simulink model "STEVE_Simulation"  (R2025b)
settings: Solver=ode8  StartTime=0  StopTime=300  FixedStep=0.0001  MaxStep=0.0001  RelTol=1e-3
model workspace (MAT data in the model file):
  op_trim1 : opcond.OperatingReport (value not decoded)
undefined symbols (not defined in the file): a_gyro_fast, Actuators, AeroData, b_gyro_fast, C_inner_launch_d_Kd, C_inner_launch_d_Ki, C_inner_launch_d_Kp, C_inner_maxQ_d_Kd, C_inner_maxQ_d_Ki, C_inner_maxQ_d_Kp, C_inner_maxQ_d_Tf, C_outer_launch_d_Kd, C_outer_launch_d_Ki, C_outer_launch_d_Kp, C_outer_launch_d_N, C_outer_maxQ_d_Kd, C_outer_maxQ_d_Ki, C_outer_maxQ_d_Kp, dspblkCoreblockFVToolHelper, F, fractalcoef, fs_filter, fs_gyro, gcbh, Initial, K_gains, Light, max_q_margin, MIL, PrelookupData, Ref_Area, rocket_length, RocketAeroPhysical, time_vector, timeStep, Ts_inner, Ts_outer, wn_ramp
libraries: simulink x14, simulink_extras x11, slpidlib x10, aerolibwind2 x3, aerolibasang x3, aerolibtransform2 x2, aerolibatmos2 x1, sensorgpslib x1, mspsensorlib x1, aerolibconvert2 x1, aerolibactuator x1
(part 2 of 3)

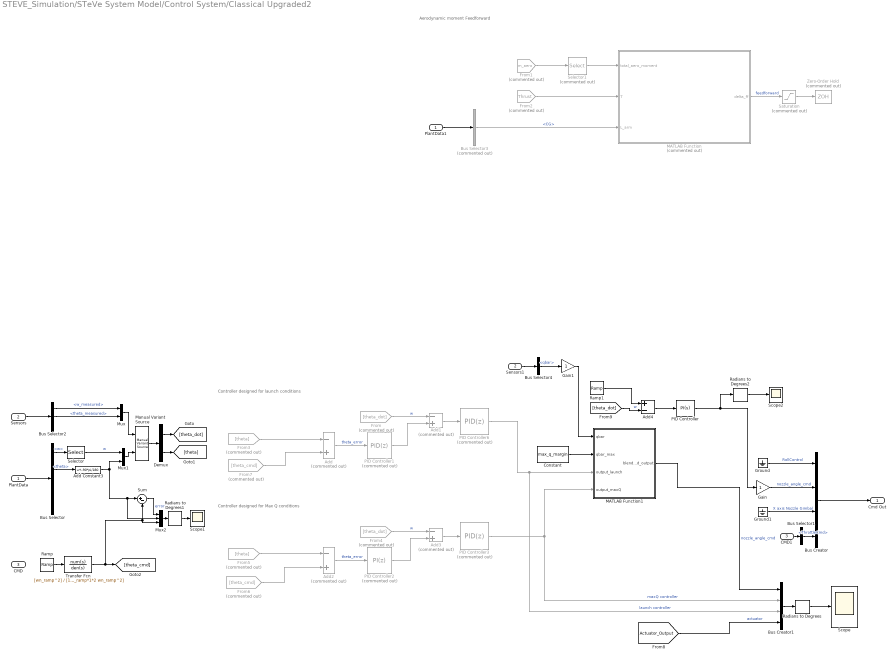
== system STEVE_Simulation/STeVe System Model/Control System/Classical Upgraded2 ==
  note: Controller designed for launch conditions
  note: Aerodynamic moment Feedforward
  note: Controller designed for Max Q conditions
  PlantData : Inport
  Sensors : Inport  Port=2
  CMD : Inport  Port=3
  Add{,1..3} (4 alike) : Sum  Commented=on  Inputs=-+
  Add Constant3 : Bias  Bias=-90*pi/180  SaturateOnIntegerOverflow=off
  Add4 : Sum  Inputs=+-
  Bus Creator : BusCreator  Inputs=4
  Bus Creator1 : BusCreator  Inputs=4
  Bus Selector : BusSelector  OutputSignals=w,body angles.theta,Ve,Xe
  Bus Selector1 : BusSelector  OutputSignals=ThrottleCmd
  Bus Selector2 : BusSelector  OutputSignals=w_measured,theta_measured,qbar
  Bus Selector3 : BusSelector  Commented=on  OutputSignals=CG
  Bus Selector4 : BusSelector  OutputSignals=qbar
  CMD1 : InportShadow  Port=3
  Constant : Constant  Value=max_q_margin
  Demux : Demux  Outputs=2
  From : From  Commented=on  GotoTag=theta_dot
  From1 : From  Commented=on  GotoTag=m_aero  TagVisibility=global
  From2 : From  Commented=on  GotoTag=Thrust  TagVisibility=global
  From3 : From  Commented=on  GotoTag=theta
  From4 : From  Commented=on  GotoTag=theta_dot
  From5 : From  Commented=on  GotoTag=theta
  From6 : From  Commented=on  GotoTag=theta_cmd
  From7 : From  Commented=on  GotoTag=theta_cmd
  Gain : Gain
  Gain1 : Gain
  Ground : Ground
  Ground1 : Ground
  MATLAB Function : MATLAB Function  Commented=on  TreatAsAtomicUnit=on
  MATLAB Function1 : MATLAB Function  TreatAsAtomicUnit=on
  Manual Variant Source : simulink/Signal Routing/Manual Variant Source  NumChoices=2  LabelModeActiveChoice=V_2
  Mux : Mux  Inputs=2
  Mux1 : Mux  Inputs=2
  Mux2 : Mux  Inputs=3
  PID Controller : slpidlib/PID Controller  Controller=PI  Form=Parallel  TimeDomain=Continuous-time  UseExternalTs=off  SampleTime=1/10  IntegratorMethod=Trapezoidal  FilterMethod=Forward Euler  ControllerParametersSource=internal  P=1.8265  I=14.0169  UseKiTs=off  D=0  UseExternalDerivativeSource=off  N=100  UseFilter=on  TunerSelectOption=Transfer Function Based (PID Tuner App)  InitialConditionSource=internal  InitialConditionForIntegrator=0  InitialConditionForFilter=0  DifferentiatorICPrevScaledInput=0  ExternalReset=none  TrackingMode=off  Kt=1  LimitOutput=off  SatLimitsSource=internal  UpperSaturationLimit=inf  LowerSaturationLimit=-inf  LinearizeAsGain=on  AntiWindupMode=none  Kb=1  LimitIntegrator=off  UpperIntegratorSaturationLimit=inf  LowerIntegratorSaturationLimit=-inf  POutMin=[]  POutMax=[]  IOutMin=[]  IOutMax=[]  DOutMin=[]  DOutMax=[]  NOutMin=[]  NOutMax=[]  SumOutMin=[]  SumOutMax=[]  SaturationOutMin=[]  SaturationOutMax=[]  PParamMin=[]  PParamMax=[]  IParamMin=[]  IParamMax=[]  DParamMin=[]  DParamMax=[]  NParamMin=[]  NParamMax=[]  KbParamMin=[]  KbParamMax=[]  KtParamMin=[]  KtParamMax=[]  KbOutMin=[]  KbOutMax=[]  KtOutMin=[]  KtOutMax=[]  IntegratorOutMin=[]  IntegratorOutMax=[]  FilterOutMin=[]  FilterOutMax=[]  SumI1OutMin=[]  SumI1OutMax=[]  SumI2OutMin=[]  SumI2OutMax=[]  SumI3OutMin=[]  SumI3OutMax=[]  SumI4OutMin=[]  SumI4OutMax=[]  SumDOutMin=[]  SumDOutMax=[]  DifferentiatorOutMin=[]  DifferentiatorOutMax=[]  FilterDiffOutCoefMin=[]  FilterDiffOutCoefMax=[]  ReciprocalOutMin=[]  ReciprocalOutMax=[]  SumDenOutMin=[]  SumDenOutMax=[]  SumNumOutMin=[]  SumNumOutMax=[]  DivideOutMin=[]  DivideOutMax=[]  UdiffTsProdOutMin=[]  UdiffTsProdOutMax=[]  NTsProdOutMin=[]  NTsProdOutMax=[]  UintegralTsProdOutMin=[]  UintegralTsProdOutMax=[]  UngainTsProdOutMin=[]  UngainTsProdOutMax=[]  ClampingZeroOutDataTypeStr=Inherit: Inherit via back propagation  ClampingZeroOutMin=[]  ClampingZeroOutMax=[]  FilterDenConstantOutDataTypeStr=Inherit: Inherit via back propagation  FilterDenConstantOutMin=[]  FilterDenConstantOutMax=[]  PCopyOutDataTypeStr=Inherit: Inherit via back propagation  PCopyOutMin=[]  PCopyOutMax=[]  NCopyOutDataTypeStr=Inherit: Inherit via back propagation  NCopyOutMin=[]  NCopyOutMax=[]  IntegratorContinuousStateAttributes=''  IntegratorStateMustResolveToSignalObject=off  IntegratorRTWStateStorageClass=Auto  FilterContinuousStateAttributes=''  FilterStateMustResolveToSignalObject=off  FilterRTWStateStorageClass=Auto  ParallelPVariant=InternalParameters  IdealPVariant=Disabled  IVariant=InternalParameters  DVariant=Disabled  IntegratorVariant=Continuous  SatVariant=Disabled  AWVariant=Passthrough  PCopyVariant=Disabled  TRVariant=Disabled  FdbkBlocksVariant=Forward  IdealPFdbkVariant=Disabled  SatFdbkVariant=Disabled  DerivativeFilterVariant=Disabled  NVariant=Disabled  NCopyVariant=Disabled_SignalSpec  FilterICVariant=Disabled  IntegratorICVariant=InternalICs  ExternalResetVariant=Disabled  TRSumVariant=Passthrough  SumFdbkVariant=Disabled  SumVariant=Sum_PI  TsampFilterVariant=InternalTs  TsampNgainVariant=Passthrough  TsampIntegralVariant=Disabled_SignalSpec  ExternalSaturationOutDataTypeStr=Inherit: Same as second input  DerivativeSourceVariant=Disabled  PreIntVariant=InternalPreInt
  PID Controller1 : slpidlib/PID Controller  Commented=on  Controller=PID  Form=Parallel  TimeDomain=Discrete-time  UseExternalTs=off  SampleTime=Ts_outer  IntegratorMethod=Forward Euler  FilterMethod=Forward Euler  ControllerParametersSource=internal  P=C_outer_launch_d_Kp  I=C_outer_launch_d_Ki  UseKiTs=off  D=C_outer_launch_d_Kd  UseExternalDerivativeSource=off  N=C_outer_launch_d_N  UseFilter=on  TunerSelectOption=Transfer Function Based (PID Tuner App)  InitialConditionSource=internal  InitialConditionForIntegrator=0  InitialConditionForFilter=0  DifferentiatorICPrevScaledInput=0  ExternalReset=none  TrackingMode=off  Kt=1  LimitOutput=off  SatLimitsSource=internal  UpperSaturationLimit=inf  LowerSaturationLimit=-inf  LinearizeAsGain=on  AntiWindupMode=none  Kb=1  LimitIntegrator=off  UpperIntegratorSaturationLimit=inf  LowerIntegratorSaturationLimit=-inf  POutMin=[]  POutMax=[]  IOutMin=[]  IOutMax=[]  DOutMin=[]  DOutMax=[]  NOutMin=[]  NOutMax=[]  SumOutMin=[]  SumOutMax=[]  SaturationOutMin=[]  SaturationOutMax=[]  PParamMin=[]  PParamMax=[]  IParamMin=[]  IParamMax=[]  DParamMin=[]  DParamMax=[]  NParamMin=[]  NParamMax=[]  KbParamMin=[]  KbParamMax=[]  KtParamMin=[]  KtParamMax=[]  KbOutMin=[]  KbOutMax=[]  KtOutMin=[]  KtOutMax=[]  IntegratorOutMin=[]  IntegratorOutMax=[]  FilterOutMin=[]  FilterOutMax=[]  SumI1OutMin=[]  SumI1OutMax=[]  SumI2OutMin=[]  SumI2OutMax=[]  SumI3OutMin=[]  SumI3OutMax=[]  SumI4OutMin=[]  SumI4OutMax=[]  SumDOutMin=[]  SumDOutMax=[]  DifferentiatorOutMin=[]  DifferentiatorOutMax=[]  FilterDiffOutCoefMin=[]  FilterDiffOutCoefMax=[]  ReciprocalOutMin=[]  ReciprocalOutMax=[]  SumDenOutMin=[]  SumDenOutMax=[]  SumNumOutMin=[]  SumNumOutMax=[]  DivideOutMin=[]  DivideOutMax=[]  UdiffTsProdOutMin=[]  UdiffTsProdOutMax=[]  NTsProdOutMin=[]  NTsProdOutMax=[]  UintegralTsProdOutMin=[]  UintegralTsProdOutMax=[]  UngainTsProdOutMin=[]  UngainTsProdOutMax=[]  ClampingZeroOutDataTypeStr=Inherit: Inherit via back propagation  ClampingZeroOutMin=[]  ClampingZeroOutMax=[]  FilterDenConstantOutDataTypeStr=Inherit: Inherit via back propagation  FilterDenConstantOutMin=[]  FilterDenConstantOutMax=[]  PCopyOutDataTypeStr=Inherit: Inherit via back propagation  PCopyOutMin=[]  PCopyOutMax=[]  NCopyOutDataTypeStr=Inherit: Inherit via back propagation  NCopyOutMin=[]  NCopyOutMax=[]  IntegratorContinuousStateAttributes=''  IntegratorStateMustResolveToSignalObject=off  IntegratorRTWStateStorageClass=Auto  FilterContinuousStateAttributes=''  FilterStateMustResolveToSignalObject=off  FilterRTWStateStorageClass=Auto  ParallelPVariant=InternalParameters  IdealPVariant=Disabled  IVariant=InternalParameters  DVariant=InternalParameters  IntegratorVariant=Discrete  SatVariant=Disabled  AWVariant=Passthrough  PCopyVariant=Disabled  TRVariant=Disabled  FdbkBlocksVariant=Forward  IdealPFdbkVariant=Disabled  SatFdbkVariant=Disabled  DerivativeFilterVariant=ForwardEulerFilter  NVariant=InternalParameters  NCopyVariant=Disabled  FilterICVariant=InternalICsFilter  IntegratorICVariant=InternalICs  ExternalResetVariant=Disabled  TRSumVariant=Passthrough  SumFdbkVariant=Disabled  SumVariant=Sum_PID  TsampFilterVariant=InternalTs  TsampNgainVariant=Passthrough  TsampIntegralVariant=Disabled_SignalSpec  ExternalSaturationOutDataTypeStr=Inherit: Same as second input  DerivativeSourceVariant=ErrorSignal  PreIntVariant=InternalPreInt
  PID Controller2 : slpidlib/PID Controller  Commented=on  Controller=PI  Form=Parallel  TimeDomain=Discrete-time  UseExternalTs=off  SampleTime=Ts_outer  IntegratorMethod=Forward Euler  FilterMethod=Forward Euler  ControllerParametersSource=internal  P=C_outer_maxQ_d_Kp  I=C_outer_maxQ_d_Ki  UseKiTs=off  D=C_outer_maxQ_d_Kd  UseExternalDerivativeSource=off  N=3.44088549948957  UseFilter=off  TunerSelectOption=Transfer Function Based (PID Tuner App)  InitialConditionSource=internal  InitialConditionForIntegrator=0  InitialConditionForFilter=0  DifferentiatorICPrevScaledInput=0  ExternalReset=none  TrackingMode=off  Kt=1  LimitOutput=off  SatLimitsSource=internal  UpperSaturationLimit=inf  LowerSaturationLimit=-inf  LinearizeAsGain=on  AntiWindupMode=none  Kb=1  LimitIntegrator=off  UpperIntegratorSaturationLimit=inf  LowerIntegratorSaturationLimit=-inf  POutMin=[]  POutMax=[]  IOutMin=[]  IOutMax=[]  DOutMin=[]  DOutMax=[]  NOutMin=[]  NOutMax=[]  SumOutMin=[]  SumOutMax=[]  SaturationOutMin=[]  SaturationOutMax=[]  PParamMin=[]  PParamMax=[]  IParamMin=[]  IParamMax=[]  DParamMin=[]  DParamMax=[]  NParamMin=[]  NParamMax=[]  KbParamMin=[]  KbParamMax=[]  KtParamMin=[]  KtParamMax=[]  KbOutMin=[]  KbOutMax=[]  KtOutMin=[]  KtOutMax=[]  IntegratorOutMin=[]  IntegratorOutMax=[]  FilterOutMin=[]  FilterOutMax=[]  SumI1OutMin=[]  SumI1OutMax=[]  SumI2OutMin=[]  SumI2OutMax=[]  SumI3OutMin=[]  SumI3OutMax=[]  SumI4OutMin=[]  SumI4OutMax=[]  SumDOutMin=[]  SumDOutMax=[]  DifferentiatorOutMin=[]  DifferentiatorOutMax=[]  FilterDiffOutCoefMin=[]  FilterDiffOutCoefMax=[]  ReciprocalOutMin=[]  ReciprocalOutMax=[]  SumDenOutMin=[]  SumDenOutMax=[]  SumNumOutMin=[]  SumNumOutMax=[]  DivideOutMin=[]  DivideOutMax=[]  UdiffTsProdOutMin=[]  UdiffTsProdOutMax=[]  NTsProdOutMin=[]  NTsProdOutMax=[]  UintegralTsProdOutMin=[]  UintegralTsProdOutMax=[]  UngainTsProdOutMin=[]  UngainTsProdOutMax=[]  ClampingZeroOutDataTypeStr=Inherit: Inherit via back propagation  ClampingZeroOutMin=[]  ClampingZeroOutMax=[]  FilterDenConstantOutDataTypeStr=Inherit: Inherit via back propagation  FilterDenConstantOutMin=[]  FilterDenConstantOutMax=[]  PCopyOutDataTypeStr=Inherit: Inherit via back propagation  PCopyOutMin=[]  PCopyOutMax=[]  NCopyOutDataTypeStr=Inherit: Inherit via back propagation  NCopyOutMin=[]  NCopyOutMax=[]  IntegratorContinuousStateAttributes=''  IntegratorStateMustResolveToSignalObject=off  IntegratorRTWStateStorageClass=Auto  FilterContinuousStateAttributes=''  FilterStateMustResolveToSignalObject=off  FilterRTWStateStorageClass=Auto  ParallelPVariant=InternalParameters  IdealPVariant=Disabled  IVariant=InternalParameters  DVariant=Disabled  IntegratorVariant=Discrete  SatVariant=Disabled  AWVariant=Passthrough  PCopyVariant=Disabled  TRVariant=Disabled  FdbkBlocksVariant=Forward  IdealPFdbkVariant=Disabled  SatFdbkVariant=Disabled  DerivativeFilterVariant=Disabled  NVariant=Disabled  NCopyVariant=Disabled_SignalSpec  FilterICVariant=Disabled  IntegratorICVariant=InternalICs  ExternalResetVariant=Disabled  TRSumVariant=Passthrough  SumFdbkVariant=Disabled  SumVariant=Sum_PI  TsampFilterVariant=InternalTs  TsampNgainVariant=Passthrough  TsampIntegralVariant=Disabled_SignalSpec  ExternalSaturationOutDataTypeStr=Inherit: Same as second input  DerivativeSourceVariant=Disabled  PreIntVariant=InternalPreInt
  PID Controller3 : slpidlib/PID Controller  Commented=on  Controller=PID  Form=Parallel  TimeDomain=Discrete-time  UseExternalTs=off  SampleTime=Ts_inner  IntegratorMethod=Forward Euler  FilterMethod=Forward Euler  ControllerParametersSource=internal  P=C_inner_maxQ_d_Kp  I=C_inner_maxQ_d_Ki  UseKiTs=off  D=C_inner_maxQ_d_Kd  UseExternalDerivativeSource=off  N=C_inner_maxQ_d_Tf  UseFilter=on  TunerSelectOption=Transfer Function Based (PID Tuner App)  InitialConditionSource=internal  InitialConditionForIntegrator=0  InitialConditionForFilter=0  DifferentiatorICPrevScaledInput=0  ExternalReset=none  TrackingMode=off  Kt=1  LimitOutput=on  SatLimitsSource=internal  UpperSaturationLimit=10*pi/180  LowerSaturationLimit=-10*pi/180  LinearizeAsGain=on  AntiWindupMode=clamping  Kb=1  LimitIntegrator=on  UpperIntegratorSaturationLimit=10*pi/180  LowerIntegratorSaturationLimit=-10*pi/180  POutMin=[]  POutMax=[]  IOutMin=[]  IOutMax=[]  DOutMin=[]  DOutMax=[]  NOutMin=[]  NOutMax=[]  SumOutMin=[]  SumOutMax=[]  SaturationOutMin=[]  SaturationOutMax=[]  PParamMin=[]  PParamMax=[]  IParamMin=[]  IParamMax=[]  DParamMin=[]  DParamMax=[]  NParamMin=[]  NParamMax=[]  KbParamMin=[]  KbParamMax=[]  KtParamMin=[]  KtParamMax=[]  KbOutMin=[]  KbOutMax=[]  KtOutMin=[]  KtOutMax=[]  IntegratorOutMin=[]  IntegratorOutMax=[]  FilterOutMin=[]  FilterOutMax=[]  SumI1OutMin=[]  SumI1OutMax=[]  SumI2OutMin=[]  SumI2OutMax=[]  SumI3OutMin=[]  SumI3OutMax=[]  SumI4OutMin=[]  SumI4OutMax=[]  SumDOutMin=[]  SumDOutMax=[]  DifferentiatorOutMin=[]  DifferentiatorOutMax=[]  FilterDiffOutCoefMin=[]  FilterDiffOutCoefMax=[]  ReciprocalOutMin=[]  ReciprocalOutMax=[]  SumDenOutMin=[]  SumDenOutMax=[]  SumNumOutMin=[]  SumNumOutMax=[]  DivideOutMin=[]  DivideOutMax=[]  UdiffTsProdOutMin=[]  UdiffTsProdOutMax=[]  NTsProdOutMin=[]  NTsProdOutMax=[]  UintegralTsProdOutMin=[]  UintegralTsProdOutMax=[]  UngainTsProdOutMin=[]  UngainTsProdOutMax=[]  ClampingZeroOutDataTypeStr=Inherit: Inherit via back propagation  ClampingZeroOutMin=[]  ClampingZeroOutMax=[]  FilterDenConstantOutDataTypeStr=Inherit: Inherit via back propagation  FilterDenConstantOutMin=[]  FilterDenConstantOutMax=[]  PCopyOutDataTypeStr=Inherit: Inherit via back propagation  PCopyOutMin=[]  PCopyOutMax=[]  NCopyOutDataTypeStr=Inherit: Inherit via back propagation  NCopyOutMin=[]  NCopyOutMax=[]  IntegratorContinuousStateAttributes=''  IntegratorStateMustResolveToSignalObject=off  IntegratorRTWStateStorageClass=Auto  FilterContinuousStateAttributes=''  FilterStateMustResolveToSignalObject=off  FilterRTWStateStorageClass=Auto  ParallelPVariant=InternalParameters  IdealPVariant=Disabled  IVariant=InternalParameters  DVariant=InternalParameters  IntegratorVariant=Discrete  SatVariant=Enabled  AWVariant=DiscClampingParallel  PCopyVariant=Disabled  TRVariant=Disabled  FdbkBlocksVariant=Forward  IdealPFdbkVariant=Disabled  SatFdbkVariant=Disabled  DerivativeFilterVariant=ForwardEulerFilter  NVariant=InternalParameters  NCopyVariant=Disabled  FilterICVariant=InternalICsFilter  IntegratorICVariant=InternalICs  ExternalResetVariant=Disabled  TRSumVariant=Passthrough  SumFdbkVariant=Disabled  SumVariant=Sum_PID  TsampFilterVariant=InternalTs  TsampNgainVariant=Passthrough  TsampIntegralVariant=Disabled_SignalSpec  ExternalSaturationOutDataTypeStr=Inherit: Same as second input  DerivativeSourceVariant=ErrorSignal  PreIntVariant=InternalPreInt
  PID Controller6 : slpidlib/PID Controller  Commented=on  Controller=PID  Form=Parallel  TimeDomain=Discrete-time  UseExternalTs=off  SampleTime=Ts_inner  IntegratorMethod=Forward Euler  FilterMethod=Forward Euler  ControllerParametersSource=internal  P=C_inner_launch_d_Kp  I=C_inner_launch_d_Ki  UseKiTs=off  D=C_inner_launch_d_Kd  UseExternalDerivativeSource=off  N=100  UseFilter=off  TunerSelectOption=Transfer Function Based (PID Tuner App)  InitialConditionSource=internal  InitialConditionForIntegrator=0  InitialConditionForFilter=0  DifferentiatorICPrevScaledInput=0  ExternalReset=none  TrackingMode=off  Kt=1  LimitOutput=on  SatLimitsSource=internal  UpperSaturationLimit=10*pi/180  LowerSaturationLimit=-10*pi/180  LinearizeAsGain=on  AntiWindupMode=clamping  Kb=1  LimitIntegrator=on  UpperIntegratorSaturationLimit=10*pi/180  LowerIntegratorSaturationLimit=-10*pi/180  POutMin=[]  POutMax=[]  IOutMin=[]  IOutMax=[]  DOutMin=[]  DOutMax=[]  NOutMin=[]  NOutMax=[]  SumOutMin=[]  SumOutMax=[]  SaturationOutMin=[]  SaturationOutMax=[]  PParamMin=[]  PParamMax=[]  IParamMin=[]  IParamMax=[]  DParamMin=[]  DParamMax=[]  NParamMin=[]  NParamMax=[]  KbParamMin=[]  KbParamMax=[]  KtParamMin=[]  KtParamMax=[]  KbOutMin=[]  KbOutMax=[]  KtOutMin=[]  KtOutMax=[]  IntegratorOutMin=[]  IntegratorOutMax=[]  FilterOutMin=[]  FilterOutMax=[]  SumI1OutMin=[]  SumI1OutMax=[]  SumI2OutMin=[]  SumI2OutMax=[]  SumI3OutMin=[]  SumI3OutMax=[]  SumI4OutMin=[]  SumI4OutMax=[]  SumDOutMin=[]  SumDOutMax=[]  DifferentiatorOutMin=[]  DifferentiatorOutMax=[]  FilterDiffOutCoefMin=[]  FilterDiffOutCoefMax=[]  ReciprocalOutMin=[]  ReciprocalOutMax=[]  SumDenOutMin=[]  SumDenOutMax=[]  SumNumOutMin=[]  SumNumOutMax=[]  DivideOutMin=[]  DivideOutMax=[]  UdiffTsProdOutMin=[]  UdiffTsProdOutMax=[]  NTsProdOutMin=[]  NTsProdOutMax=[]  UintegralTsProdOutMin=[]  UintegralTsProdOutMax=[]  UngainTsProdOutMin=[]  UngainTsProdOutMax=[]  ClampingZeroOutDataTypeStr=Inherit: Inherit via back propagation  ClampingZeroOutMin=[]  ClampingZeroOutMax=[]  FilterDenConstantOutDataTypeStr=Inherit: Inherit via back propagation  FilterDenConstantOutMin=[]  FilterDenConstantOutMax=[]  PCopyOutDataTypeStr=Inherit: Inherit via back propagation  PCopyOutMin=[]  PCopyOutMax=[]  NCopyOutDataTypeStr=Inherit: Inherit via back propagation  NCopyOutMin=[]  NCopyOutMax=[]  IntegratorContinuousStateAttributes=''  IntegratorStateMustResolveToSignalObject=off  IntegratorRTWStateStorageClass=Auto  FilterContinuousStateAttributes=''  FilterStateMustResolveToSignalObject=off  FilterRTWStateStorageClass=Auto  ParallelPVariant=InternalParameters  IdealPVariant=Disabled  IVariant=InternalParameters  DVariant=InternalParameters  IntegratorVariant=Discrete  SatVariant=Enabled  AWVariant=DiscClampingParallel  PCopyVariant=Disabled  TRVariant=Disabled  FdbkBlocksVariant=Forward  IdealPFdbkVariant=Disabled  SatFdbkVariant=Disabled  DerivativeFilterVariant=Differentiator  NVariant=Passthrough  NCopyVariant=Disabled_SignalSpec  FilterICVariant=InternalICsDifferentiator  IntegratorICVariant=InternalICs  ExternalResetVariant=Disabled  TRSumVariant=Passthrough  SumFdbkVariant=Disabled  SumVariant=Sum_PID  TsampFilterVariant=InternalTs  TsampNgainVariant=Passthrough  TsampIntegralVariant=Disabled_SignalSpec  ExternalSaturationOutDataTypeStr=Inherit: Same as second input  DerivativeSourceVariant=ErrorSignal  PreIntVariant=InternalPreInt
  PlantData1 : InportShadow
  Radians to Degrees : simulink_extras/Transformations/Radians to Degrees
  Radians to Degrees1 : simulink_extras/Transformations/Radians to Degrees
  Radians to Degrees2 : simulink_extras/Transformations/Radians to Degrees
  Ramp : simulink/Sources/Ramp  slope=-(50/60)*pi/180  start=0  InitialOutput=0
  Ramp1 : simulink/Sources/Ramp  slope=0  start=0  InitialOutput=0
  Saturation : Saturate  Commented=on  UpperLimit=10*pi/180  LowerLimit=-10*pi/180
  Scope : Scope
      settings: ActiveDisplayYMinimum=-0.083485750616447252  ActiveDisplayYMaximum=2.7048040540539371  DataLoggingVariableName=ScopeData3
  Scope1 : Scope
      settings: ActiveDisplayYMinimum=-44.397461498284216  ActiveDisplayYMaximum=2.337544107445984  DataLoggingVariableName=ScopeData4
  Scope2 : Scope
      settings: ActiveDisplayYMinimum=-0.57661888935781047  ActiveDisplayYMaximum=0.0662657690157187  DataLoggingVariableName=ScopeData9
  Selector : Selector  InputPortWidth=3  IndexOptions=Index vector (dialog)  Indices=[2]  OutputSizes=1
  Selector1 : Selector  Commented=on  InputPortWidth=3  IndexOptions=Index vector (dialog)  Indices=[2]  OutputSizes=1
  Sensors1 : InportShadow  Port=2
  Sum : Sum  Inputs=|+-
  Transfer Fcn : TransferFcn  Numerator=[wn_ramp^2]  Denominator=[1 wn_ramp*1*2 wn_ramp^2]
  Zero-Order Hold : ZeroOrderHold  Commented=on  SampleTime=0.005
  Cmd Out : Outport
  wires:
  Selector1/1 -> MATLAB Function/1(total_aero_moment)
  PlantData/1 -> Bus Selector/1
  From1/1 -> Selector1/1
  Bus Selector/1 -> Selector/1  "<w>"
  Ground1/1 -> Bus Creator/3  "X axis Nozzle Gimbal"
  Bus Selector3/1 -> MATLAB Function/3(L_arm)  "<CG>"
  Gain/1 -> Bus Creator/2  "nozzle_angle_cmd"
  MATLAB Function/1(delta_ff) -> Saturation/1  "feedforward"
  From/1 -> Add1/1  "w"
  PlantData1/1 -> Bus Selector3/1
  From7/1 -> Add/2
  Ground/1 -> Bus Creator/1  "RollControl"
  From2/1 -> MATLAB Function/2(T)
  Bus Creator/1 -> Cmd Out/1
  Add/1 -> PID Controller1/1  "theta_error"
  PID Controller6/1 -> Bus Creator1/3, MATLAB Function1/3(output_launch)  "launch controller"
  Add1/1 -> PID Controller6/1
  Sensors/1 -> Bus Selector2/1
  Saturation/1 -> Zero-Order Hold/1
  From3/1 -> Add/1
  CMD1/1 -> Bus Selector1/1
  Bus Selector1/1 -> Bus Creator/4  "<ThrottleCmd>"
  PID Controller1/1 -> Add1/2
  Bus Selector/2 -> Add Constant3/1  "<theta>"
  Add2/1 -> PID Controller2/1  "theta_error"
  From5/1 -> Add2/1
  Add3/1 -> PID Controller3/1
  PID Controller3/1 -> Bus Creator1/2, MATLAB Function1/4(output_maxQ)  "maxQ controller"
  PID Controller2/1 -> Add3/2
  From6/1 -> Add2/2
  From4/1 -> Add3/1  "w"
  Ramp/1 -> Transfer Fcn/1
  Sensors1/1 -> Bus Selector4/1
  MATLAB Function1/1(blended_output) -> Bus Creator1/1  "nozzle_angle_cmd"
  Constant/1 -> MATLAB Function1/2(qbar_max)
  Bus Selector4/1 -> Gain1/1  "<qbar>"
  [Actuator_Output] -> Bus Creator1/4  "actuator"
  Transfer Fcn/1 -> Mux2/3, Sum/2, [theta_cmd]
  Bus Selector2/1 -> Mux/1  "<w_measured>"
  Bus Selector2/2 -> Mux/2  "<theta_measured>"
  Mux/1 -> Manual Variant Source/1
  Manual Variant Source/1 -> Demux/1
  Demux/1 -> [theta_dot]
  Demux/2 -> [theta]
  Selector/1 -> Mux1/1  "w"
  Mux1/1 -> Manual Variant Source/2
  Add Constant3/1 -> Mux2/2, Sum/1, Mux1/2
  Sum/1 -> Mux2/1  "error"
  Gain1/1 -> MATLAB Function1/1(qbar)
  Bus Creator1/1 -> Radians to Degrees/1
  Radians to Degrees/1 -> Scope/1
  Mux2/1 -> Radians to Degrees1/1
  Radians to Degrees1/1 -> Scope1/1
  [theta_dot] -> Add4/2  "w"
  Add4/1 -> PID Controller/1
  Ramp1/1 -> Add4/1
  PID Controller/1 -> Radians to Degrees2/1, Gain/1
  Radians to Degrees2/1 -> Scope2/1

== system STEVE_Simulation/STeVe System Model/Control System/ControlSystem Classical ==
  note: FeedForward Controller
  AvionicsBus : Inport
  Guidance : Inport  Port=2
  Add : Sum
  Bus Creator : BusCreator  Inputs=4
  Bus Selector : BusSelector  OutputSignals=ThetaCmd,ThrottleCmd
  Bus Selector1 : BusSelector  OutputSignals=w,body angles.theta
  Constant : Constant  Value=Actuators.Engine.MaxThrust
  Constant1 : Constant  Value=4
  Ground : Ground
  Ground1 : Ground
  Integrator : Integrator
  Multiply : Gain
  Multiply1 : Gain  Gain=0.1
  Multiply2 : Gain  Gain=-1
  Multiply3 : Gain
  Multiply4 : Gain  Gain=0.05
  Product : Product
  Product1 : Product  Inputs=*/
  Selector : Selector  InputPortWidth=3  IndexOptions=Index vector (dialog)  Indices=2  OutputSizes=1
  Selector1 : Selector  InputPortWidth=3  IndexOptions=Index vector (dialog)  Indices=[2]  OutputSizes=1
  Sum : Sum  Inputs=-+|
  Sum1 : Sum  Inputs=-|+|+
  Sum2 : Sum  Inputs=|++
  cmd : Outport
  wires:
  Bus Creator/1 -> cmd/1
  Ground/1 -> Bus Creator/1  "RollControl"
  Ground1/1 -> Bus Creator/3  "X axis Nozzle Gimbal"
  Guidance/1 -> Bus Selector/1
  Bus Selector/2 -> Bus Creator/4  "<ThrottleCmd>"
  Bus Selector/1 -> Sum/2  "<ThetaCmd>"
  AvionicsBus/1 -> Bus Selector1/1
  Bus Selector1/1 -> Selector/1  "<w>"
  Multiply/1 -> Bus Creator/2  "nozzle_angle_cmd"
  Sum1/1 -> Integrator/1, Multiply1/1  "thetadot_error"
  Selector/1 -> Sum1/1  "thetadot"
  Bus Selector1/2 -> Sum/1  "<theta>"
  Sum/1 -> Multiply3/1  "theta_error"
  Constant1/1 -> Product/2
  Constant/1 -> Product/1
  Product/1 -> Product1/2
  [m_aero] -> Selector1/1
  Selector1/1 -> Product1/1
  Add/1 -> Multiply/1  "total_nozzle_angle_rad"
  Product1/1 -> Multiply2/1
  Multiply3/1 -> Sum1/2  "pitch_controller_cmd"
  Sum2/1 -> Add/2  "pitchrate_controller_cmd"
  Multiply2/1 -> Add/1  "feedforward_cmd"
  Multiply1/1 -> Sum2/1
  Integrator/1 -> Multiply4/1
  Multiply4/1 -> Sum2/2

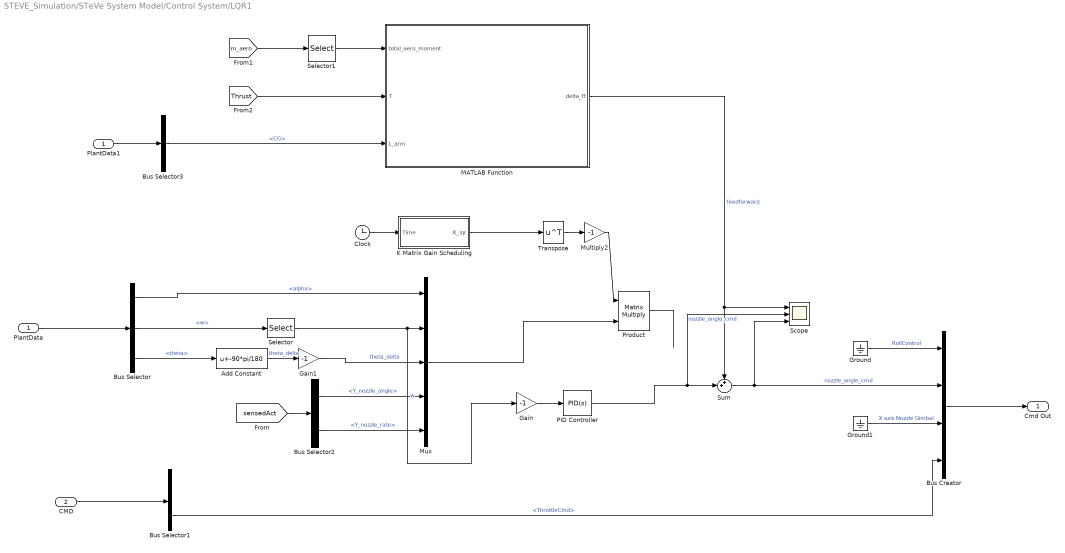
== system STEVE_Simulation/STeVe System Model/Control System/LQR1 ==
  PlantData : Inport
  CMD : Inport  Port=2
  Add Constant : Bias  Bias=-90*pi/180  SaturateOnIntegerOverflow=off
  Bus Creator : BusCreator  Inputs=4
  Bus Selector : BusSelector  OutputSignals=alpha,w,body angles.theta
  Bus Selector1 : BusSelector  OutputSignals=ThetaCmd,ThrottleCmd
  Bus Selector2 : BusSelector  OutputSignals=Y_nozzle_angle,Y_nozzle_rate
  Bus Selector3 : BusSelector  OutputSignals=CG
  Clock : Clock
  Gain : Gain  Gain=-1
  Gain1 : Gain  Gain=-1
  Ground : Ground
  Ground1 : Ground
  K Matrix Gain Scheduling : Subsystem
  MATLAB Function : MATLAB Function  TreatAsAtomicUnit=on
  Multiply2 : Gain  Gain=-1
  Mux : Mux  Inputs=5
  PID Controller : slpidlib/PID Controller  Controller=PID  Form=Parallel  TimeDomain=Continuous-time  UseExternalTs=off  SampleTime=-1  IntegratorMethod=Forward Euler  FilterMethod=Forward Euler  ControllerParametersSource=internal  P=0.00297430815475411  I=0.00270872553316802  UseKiTs=off  D=0.00015125727616714  UseExternalDerivativeSource=off  N=19.0953356399636  UseFilter=on  TunerSelectOption=Transfer Function Based (PID Tuner App)  InitialConditionSource=internal  InitialConditionForIntegrator=0  InitialConditionForFilter=0  DifferentiatorICPrevScaledInput=0  ExternalReset=none  TrackingMode=off  Kt=1  LimitOutput=off  SatLimitsSource=internal  UpperSaturationLimit=inf  LowerSaturationLimit=-inf  LinearizeAsGain=on  AntiWindupMode=none  Kb=1  LimitIntegrator=off  UpperIntegratorSaturationLimit=inf  LowerIntegratorSaturationLimit=-inf  POutMin=[]  POutMax=[]  IOutMin=[]  IOutMax=[]  DOutMin=[]  DOutMax=[]  NOutMin=[]  NOutMax=[]  SumOutMin=[]  SumOutMax=[]  SaturationOutMin=[]  SaturationOutMax=[]  PParamMin=[]  PParamMax=[]  IParamMin=[]  IParamMax=[]  DParamMin=[]  DParamMax=[]  NParamMin=[]  NParamMax=[]  KbParamMin=[]  KbParamMax=[]  KtParamMin=[]  KtParamMax=[]  KbOutMin=[]  KbOutMax=[]  KtOutMin=[]  KtOutMax=[]  IntegratorOutMin=[]  IntegratorOutMax=[]  FilterOutMin=[]  FilterOutMax=[]  SumI1OutMin=[]  SumI1OutMax=[]  SumI2OutMin=[]  SumI2OutMax=[]  SumI3OutMin=[]  SumI3OutMax=[]  SumI4OutMin=[]  SumI4OutMax=[]  SumDOutMin=[]  SumDOutMax=[]  DifferentiatorOutMin=[]  DifferentiatorOutMax=[]  FilterDiffOutCoefMin=[]  FilterDiffOutCoefMax=[]  ReciprocalOutMin=[]  ReciprocalOutMax=[]  SumDenOutMin=[]  SumDenOutMax=[]  SumNumOutMin=[]  SumNumOutMax=[]  DivideOutMin=[]  DivideOutMax=[]  UdiffTsProdOutMin=[]  UdiffTsProdOutMax=[]  NTsProdOutMin=[]  NTsProdOutMax=[]  UintegralTsProdOutMin=[]  UintegralTsProdOutMax=[]  UngainTsProdOutMin=[]  UngainTsProdOutMax=[]  ClampingZeroOutDataTypeStr=Inherit: Inherit via back propagation  ClampingZeroOutMin=[]  ClampingZeroOutMax=[]  FilterDenConstantOutDataTypeStr=Inherit: Inherit via back propagation  FilterDenConstantOutMin=[]  FilterDenConstantOutMax=[]  PCopyOutDataTypeStr=Inherit: Inherit via back propagation  PCopyOutMin=[]  PCopyOutMax=[]  NCopyOutDataTypeStr=Inherit: Inherit via back propagation  NCopyOutMin=[]  NCopyOutMax=[]  IntegratorContinuousStateAttributes=''  IntegratorStateMustResolveToSignalObject=off  IntegratorRTWStateStorageClass=Auto  FilterContinuousStateAttributes=''  FilterStateMustResolveToSignalObject=off  FilterRTWStateStorageClass=Auto  ParallelPVariant=InternalParameters  IdealPVariant=Disabled  IVariant=InternalParameters  DVariant=InternalParameters  IntegratorVariant=Continuous  SatVariant=Disabled  AWVariant=Passthrough  PCopyVariant=Disabled  TRVariant=Disabled  FdbkBlocksVariant=Forward  IdealPFdbkVariant=Disabled  SatFdbkVariant=Disabled  DerivativeFilterVariant=ContFilter  NVariant=InternalParameters  NCopyVariant=Disabled  FilterICVariant=InternalICsFilter  IntegratorICVariant=InternalICs  ExternalResetVariant=Disabled  TRSumVariant=Passthrough  SumFdbkVariant=Disabled  SumVariant=Sum_PID  TsampFilterVariant=InternalTs  TsampNgainVariant=Passthrough  TsampIntegralVariant=Disabled_SignalSpec  ExternalSaturationOutDataTypeStr=Inherit: Same as second input  DerivativeSourceVariant=ErrorSignal  PreIntVariant=InternalPreInt
  PlantData1 : InportShadow
  Product : Product  Multiplication=Matrix(*)
  Scope : Scope  NumInputPorts=3
      settings: ActiveDisplayYMinimum=-10.665603461907551  ActiveDisplayYMaximum=5.7104419346533186
  Selector : Selector  InputPortWidth=3  IndexOptions=Index vector (dialog)  Indices=[2]  OutputSizes=1
  Selector1 : Selector  InputPortWidth=3  IndexOptions=Index vector (dialog)  Indices=[2]  OutputSizes=1
  Sum : Sum  Inputs=++|
  Transpose : Math  Operator=transpose
  Cmd Out : Outport
  wires:
  PlantData/1 -> Bus Selector/1
  Bus Selector2/2 -> Mux/5  "<Y_nozzle_rate>"
  Ground/1 -> Bus Creator/1  "RollControl"
  Bus Selector/2 -> Selector/1  "<w>"
  Bus Selector2/1 -> Mux/4  "<Y_nozzle_angle>"
  [sensedAct] -> Bus Selector2/1
  Bus Selector1/2 -> Bus Creator/4  "<ThrottleCmd>"
  Bus Selector/1 -> Mux/1  "<alpha>"
  Mux/1 -> Product/2
  Ground1/1 -> Bus Creator/3  "X axis Nozzle Gimbal"
  Add Constant/1 -> Gain1/1  "theta_delta"
  Bus Creator/1 -> Cmd Out/1
  Selector/1 -> Gain/1, Mux/2  "w"
  CMD/1 -> Bus Selector1/1
  Bus Selector/3 -> Add Constant/1  "<theta>"
  K Matrix Gain Scheduling/1(K_lqr) -> Transpose/1
  Clock/1 -> K Matrix Gain Scheduling/1(Time)
  Transpose/1 -> Multiply2/1
  Multiply2/1 -> Product/1
  Sum/1 -> Scope/3, Bus Creator/2  "nozzle_angle_cmd"
  Gain1/1 -> Mux/3  "theta_delta"
  PlantData1/1 -> Bus Selector3/1
  Bus Selector3/1 -> MATLAB Function/3(L_arm)  "<CG>"
  [m_aero] -> Selector1/1
  [Thrust] -> MATLAB Function/2(T)
  Selector1/1 -> MATLAB Function/1(total_aero_moment)
  Product/1 -> ?
  MATLAB Function/1(delta_ff) -> Sum/1, Scope/1  "feedforward"
  PID Controller/1 -> Scope/2, Sum/2  "nozzle_angle_cmd"
  Gain/1 -> PID Controller/1

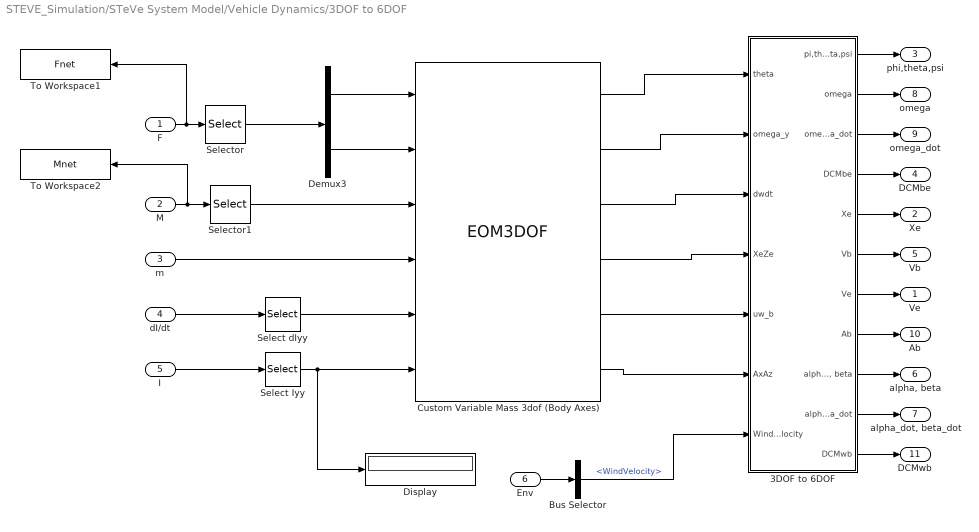
== system STEVE_Simulation/STeVe System Model/Vehicle Dynamics/3DOF to 6DOF ==
  F : Inport
  M : Inport  Port=2
  m : Inport  Port=3
  dI/dt : Inport  Port=4
  I : Inport  Port=5
  Env : Inport  Port=6
  3DOF to 6DOF : Subsystem
  Bus Selector : BusSelector  OutputSignals=WindVelocity
  Custom Variable Mass 3dof (Body Axes) : EOM3DOF  mtype=Custom Variable  v_ini=Initial.Conditions.V0  theta_ini=Initial.Conditions.theta0  pos_ini=[0 Initial.Conditions.h0]  g=0  vel_statename={'u','w'}  pos_statename={'Xe','Ze'}  q_statename='q'  theta_statename='theta'
  Demux3 : Demux  Outputs=2
  Display : Display
  Select Iyy : Selector  NumberOfDimensions=2  InputPortWidth=3  IndexOptions=Index vector (dialog),Index vector (dialog)  Indices=[2],[2]  OutputSizes=1,1
  Select dIyy : Selector  NumberOfDimensions=2  InputPortWidth=3  IndexOptions=Index vector (dialog),Index vector (dialog)  Indices=[2],[2]  OutputSizes=1,1
  Selector : Selector  InputPortWidth=3  IndexOptions=Index vector (dialog)  Indices=[1 3]  OutputSizes=1
  Selector1 : Selector  InputPortWidth=3  IndexOptions=Index vector (dialog)  Indices=[2]  OutputSizes=1
  To Workspace1 : ToWorkspace  VariableName=Fnet  SaveFormat=Timeseries  SampleTime=-1
  To Workspace2 : ToWorkspace  VariableName=Mnet  SaveFormat=Timeseries  SampleTime=-1
  Ve : Outport
  Xe : Outport  Port=2
  phi,theta,psi : Outport  Port=3
  DCMbe : Outport  Port=4
  Vb : Outport  Port=5
  "alpha, beta" : Outport  Port=6
  "alpha_dot, beta_dot" : Outport  Port=7
  omega : Outport  Port=8
  omega_dot : Outport  Port=9
  Ab : Outport  Port=10
  DCMwb : Outport  Port=11
  wires:
  F/1 -> To Workspace1/1, Selector/1
  Demux3/2 -> Custom Variable Mass 3dof (Body Axes)/2
  Demux3/1 -> Custom Variable Mass 3dof (Body Axes)/1
  Selector/1 -> Demux3/1
  M/1 -> To Workspace2/1, Selector1/1
  Selector1/1 -> Custom Variable Mass 3dof (Body Axes)/3
  Custom Variable Mass 3dof (Body Axes)/1 -> 3DOF to 6DOF/1(theta)
  Custom Variable Mass 3dof (Body Axes)/4 -> 3DOF to 6DOF/4(XeZe)
  Custom Variable Mass 3dof (Body Axes)/6 -> 3DOF to 6DOF/6(AxAz)
  3DOF to 6DOF/1(pi,theta,psi) -> phi,theta,psi/1
  3DOF to 6DOF/2(omega) -> omega/1
  3DOF to 6DOF/3(omega_dot) -> omega_dot/1
  3DOF to 6DOF/4(DCMbe) -> DCMbe/1
  3DOF to 6DOF/5(Xe) -> Xe/1
  3DOF to 6DOF/6(Vb) -> Vb/1
  3DOF to 6DOF/7(Ve) -> Ve/1
  3DOF to 6DOF/8(Ab) -> Ab/1
  3DOF to 6DOF/9("alpha, beta") -> "alpha, beta"/1
  3DOF to 6DOF/10("alpha_dot, beta_dot") -> "alpha_dot, beta_dot"/1
  I/1 -> Select Iyy/1
  dI/dt/1 -> Select dIyy/1
  m/1 -> Custom Variable Mass 3dof (Body Axes)/4
  Custom Variable Mass 3dof (Body Axes)/2 -> 3DOF to 6DOF/2(omega_y)
  Custom Variable Mass 3dof (Body Axes)/3 -> 3DOF to 6DOF/3(dwdt)
  Custom Variable Mass 3dof (Body Axes)/5 -> 3DOF to 6DOF/5(uw_b)
  Env/1 -> Bus Selector/1
  Bus Selector/1 -> 3DOF to 6DOF/7(WindVelocity)  "<WindVelocity>"
  Select dIyy/1 -> Custom Variable Mass 3dof (Body Axes)/5
  Select Iyy/1 -> Display/1, Custom Variable Mass 3dof (Body Axes)/6
  3DOF to 6DOF/11(DCMwb) -> DCMwb/1

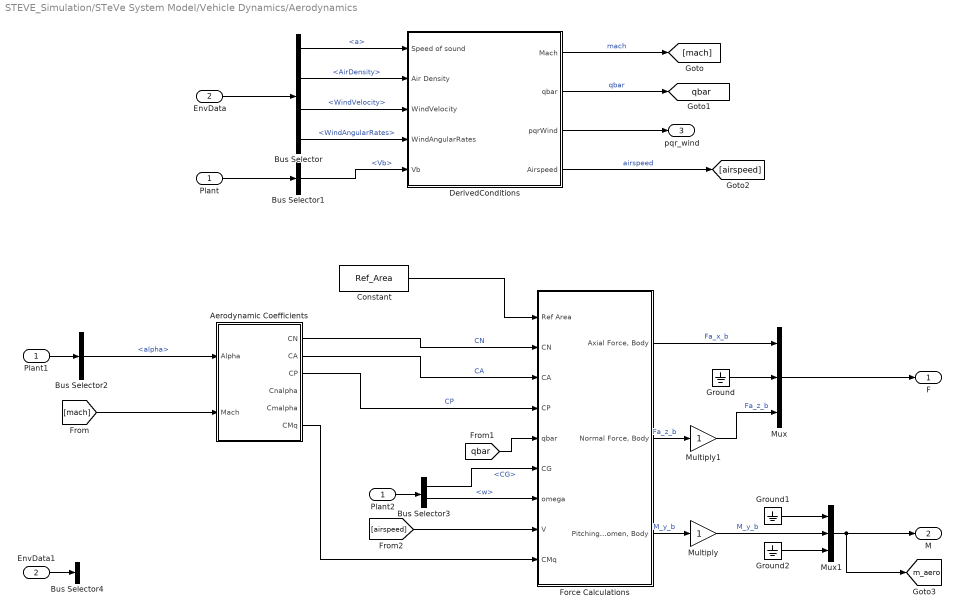
== system STEVE_Simulation/STeVe System Model/Vehicle Dynamics/Aerodynamics ==
  Plant : Inport
  EnvData : Inport  Port=2
  Aerodynamic Coefficients : Subsystem
  Bus Selector : BusSelector  OutputSignals=a,AirDensity,WindVelocity,WindAngularRates
  Bus Selector1 : BusSelector  OutputSignals=Vb
  Bus Selector2 : BusSelector  OutputSignals=alpha
  Bus Selector3 : BusSelector  OutputSignals=CG,w
  Bus Selector4 : BusSelector  OutputSignals=AirDensity
  Constant : Constant  Value=Ref_Area  VectorParams1D=off
  DerivedConditions : Subsystem
  EnvData1 : InportShadow  Port=2
  Force Calculations : Subsystem
  Ground : Ground
  Ground1 : Ground
  Ground2 : Ground
  Multiply : Gain
  Multiply1 : Gain
  Mux : Mux  Inputs=3
  Mux1 : Mux  Inputs=3
  Plant1 : InportShadow
  Plant2 : InportShadow
  F : Outport
  M : Outport  Port=2
  pqr_wind : Outport  Port=3
  tag scope: m_aero=global, qbar=global
  wires:
  Plant/1 -> Bus Selector1/1
  EnvData/1 -> Bus Selector/1
  Ground2/1 -> Mux1/3
  Ground/1 -> Mux/2
  Multiply1/1 -> Mux/3  "Fa_z_b"
  Multiply/1 -> Mux1/2  "M_y_b"
  Ground1/1 -> Mux1/1
  Force Calculations/1("Axial Force, Body") -> Mux/1  "Fa_x_b"
  Bus Selector1/1 -> DerivedConditions/5(Vb)  "<Vb>"
  Bus Selector/4 -> DerivedConditions/4(WindAngularRates)  "<WindAngularRates>"
  Bus Selector/3 -> DerivedConditions/3(WindVelocity)  "<WindVelocity>"
  Bus Selector/2 -> DerivedConditions/2(Air Density)  "<AirDensity>"
  Bus Selector/1 -> DerivedConditions/1(Speed of sound)  "<a>"
  DerivedConditions/1(Mach) -> [mach]  "mach"
  DerivedConditions/2(qbar) -> [qbar]  "qbar"
  DerivedConditions/3(pqrWind) -> pqr_wind/1
  Plant1/1 -> Bus Selector2/1
  Bus Selector2/1 -> Aerodynamic Coefficients/1(Alpha)  "<alpha>"
  [mach] -> Aerodynamic Coefficients/2(Mach)
  Constant/1 -> Force Calculations/1(Ref Area)
  Aerodynamic Coefficients/1(CN) -> Force Calculations/2(CN)  "CN"
  Aerodynamic Coefficients/2(CA) -> Force Calculations/3(CA)  "CA"
  Aerodynamic Coefficients/3(CP) -> Force Calculations/4(CP)  "CP"
  [qbar] -> Force Calculations/5(qbar)
  Plant2/1 -> Bus Selector3/1
  Bus Selector3/1 -> Force Calculations/6(CG)  "<CG>"
  Force Calculations/3("Pitching Momen, Body") -> Multiply/1  "M_y_b"
  Bus Selector3/2 -> Force Calculations/7(omega)  "<w>"
  EnvData1/1 -> Bus Selector4/1
  [airspeed] -> Force Calculations/8(V)
  Mux/1 -> F/1
  Mux1/1 -> [m_aero], M/1
  Force Calculations/2("Normal Force, Body") -> Multiply1/1  "Fa_z_b"
  Aerodynamic Coefficients/6(CMq) -> Force Calculations/9(CMq)
  DerivedConditions/4(Airspeed) -> [airspeed]  "airspeed"

== system STEVE_Simulation/STeVe System Model/Vehicle Dynamics/Propulsion F,M ==
  Actuators : Inport
  CG : Inport  Port=2
  Bus Selector : BusSelector  OutputSignals=engineThrust,Y_nozzle_angle
  Clock : Clock
  Compare To Constant : simulink/Logic and Bit Operations/Compare To Constant  relop=<  const=Actuators.Engine.BurnTime  OutDataTypeStr=boolean
  Ground : Ground
  Ground1 : Ground
  Ground2 : Ground
  Mux : Mux  Inputs=3
  Mux1 : Mux  Inputs=3
  Product : Product  OutDataTypeStr=double
  Product1 : Product  OutDataTypeStr=double
  Radians to Degrees : simulink_extras/Transformations/Radians to Degrees
  Scope : Scope
      settings: ActiveDisplayYMinimum=-2.24318  ActiveDisplayYMaximum=0.24924
  Subsystem : Subsystem
  F : Outport
  M : Outport  Port=2
  wires:
  Actuators/1 -> Bus Selector/1
  Bus Selector/2 -> Subsystem/2(Nozzle Angle), Radians to Degrees/1  "<Y_nozzle_angle>"
  Bus Selector/1 -> Subsystem/1(Thrust)  "<engineThrust>"
  Subsystem/3(M_y_b) -> Mux1/2  "M_y_b"
  Subsystem/1(Ft_x_b) -> Product/2
  Product1/1 -> Mux/3  "Ft_z_b"
  Mux/1 -> F/1
  Ground/1 -> Mux/2
  Mux1/1 -> M/1
  Ground1/1 -> Mux1/1
  Ground2/1 -> Mux1/3
  CG/1 -> Subsystem/3(CG)
  Radians to Degrees/1 -> Scope/1
  Clock/1 -> Compare To Constant/1
  Compare To Constant/1 -> Product1/1, Product/1
  Product/1 -> Mux/1  "Ft_x_b"
  Subsystem/2(Ft_z_b) -> Product1/2  "Ft_z_b"

== system STEVE_Simulation/STeVe System Model/Vehicle Dynamics/RocketEngineActuators ==
  ENV : Inport
  Commands : Inport  Port=2
  Bus Creator : BusCreator  Inputs=2
  Bus Creator1 : BusCreator  Inputs=2
  Bus Selector : BusSelector  OutputSignals=nozzle_angle_cmd,ThrottleCmd
  Bus Selector1 : BusSelector  OutputSignals=Po
  Derivative : Derivative
  MATLAB Function : MATLAB Function  TreatAsAtomicUnit=on
  Multiply : Gain
  Product : Product
  Scope : Scope  NumInputPorts=2
      settings: ActiveDisplayYMinimum=0.00020897941604108882  ActiveDisplayYMaximum=0.0026029641920276509  DataLoggingVariableName=ScopeData6
  Scope1 : Scope
      settings: ActiveDisplayYMinimum=-3298.6854275413052  ActiveDisplayYMaximum=31070.467018460706  DataLoggingVariableName=ScopeData2
  Servo : aerolibactuator/Nonlinear Second-Order Actuator  wn_fin=62  z_fin=0.5858  fin_max=10*pi/180  fin_min=-10*pi/180  fin_maxrate=(1000*pi/180)  fin_act_0=0  fin_act_vel=0
  Positions : Outport
  Sensed_Out : Outport  Port=2
  tag scope: Actuator_Output=global, Thrust=global
  wires:
  Commands/1 -> Bus Selector/1
  Bus Creator/1 -> Positions/1  "Actuators"
  Bus Selector/2 -> Product/1  "<ThrottleCmd>"
  ENV/1 -> Bus Selector1/1
  Bus Selector1/1 -> MATLAB Function/1(altitude)  "<Po>"
  MATLAB Function/1(thrust) -> Product/2
  Product/1 -> Multiply/1
  Bus Selector/1 -> Scope/1, Servo/1  "<nozzle_angle_cmd>"
  Multiply/1 -> Scope1/1, [Thrust], Bus Creator/2  "engineThrust"
  Bus Creator1/1 -> Sensed_Out/1
  Derivative/1 -> Bus Creator1/2  "Y_nozzle_rate"
  Servo/1 -> Scope/2, [Actuator_Output], Bus Creator/1  "Y_nozzle_angle"

== system STEVE_Simulation/STeVe System Model/Vehicle Dynamics/Time Varying Parameters ==
  t : Inport
  Direct Lookup Table (n-D) : LookupNDDirect  NumberOfTableDimensions=3  InputsSelectThisObjectFromTable=2-D Matrix  Table=PrelookupData.Tables.InertialTensor  DiagnosticForOutOfRangeInput=None  TableDataTypeStr=double
  Direct Lookup Table (n-D)1 : LookupNDDirect  NumberOfTableDimensions=3  InputsSelectThisObjectFromTable=2-D Matrix  Table=PrelookupData.Tables.dInertialTensor  DiagnosticForOutOfRangeInput=None  TableDataTypeStr=double
  Display : Display
  Lookup_COM_X : Interpolation_n-D  NumberOfTableDimensions=1  Table=PrelookupData.Tables.COM_X  ExtrapMethod=Clip  DiagnosticForOutOfRangeInput=Warning  RequireIndexFractionAsBus=on  InternalRulePriority=Speed
      settings: InputPortMap=u0
  Lookup_Mass : Interpolation_n-D  NumberOfTableDimensions=1  Table=PrelookupData.Tables.Mass  ExtrapMethod=Clip  DiagnosticForOutOfRangeInput=Warning  RequireIndexFractionAsBus=on  OutDataTypeStr=double  InternalRulePriority=Speed  TableDataTypeStr=Inherit: Inherit from 'Table data'
      settings: InputPortMap=u0
  Prelookup : PreLookup  BreakpointsData=PrelookupData.Breakpoints.Index  OutputSelection=Index and fraction as bus  IndexSearchMethod=Evenly spaced points
  TimeToIndex : Subsystem
  dIdt_Tensor(3x3) : Outport
  MOI_Tensor(3x3) : Outport  Port=2
  mass : Outport  Port=3
  COM_X : Outport  Port=4
  wires:
  Lookup_Mass/1 -> mass/1  "mass"
  t/1 -> TimeToIndex/1(t)
  Lookup_COM_X/1 -> COM_X/1  "CG_X"
  Direct Lookup Table (n-D)/1 -> Display/1, MOI_Tensor(3x3)/1
  Direct Lookup Table (n-D)1/1 -> dIdt_Tensor(3x3)/1
  Prelookup/1 -> Lookup_Mass/1, Lookup_COM_X/1
  TimeToIndex/1(Index) -> Direct Lookup Table (n-D)/1, Direct Lookup Table (n-D)1/1, Prelookup/1

== system STEVE_Simulation/STeVe System Model/Control System/LQR1/K Matrix Gain Scheduling ==
  Time : Inport
  1-D Lookup Table : Lookup_n-D  NumberOfTableDimensions=1  BreakpointsForDimension1=time_vector  Table=K_gains(:,1)  ExtrapMethod=Clip  InternalRulePriority=Speed  RndMeth=Simplest
  1-D Lookup Table1 : Lookup_n-D  NumberOfTableDimensions=1  BreakpointsForDimension1=time_vector  Table=K_gains(:,2)  ExtrapMethod=Clip  InternalRulePriority=Speed  RndMeth=Simplest
  1-D Lookup Table2 : Lookup_n-D  NumberOfTableDimensions=1  BreakpointsForDimension1=time_vector  Table=K_gains(:,3)  ExtrapMethod=Clip  InternalRulePriority=Speed  RndMeth=Simplest
  1-D Lookup Table3 : Lookup_n-D  NumberOfTableDimensions=1  BreakpointsForDimension1=time_vector  Table=K_gains(:,4)  ExtrapMethod=Clip  InternalRulePriority=Speed  RndMeth=Simplest
  1-D Lookup Table4 : Lookup_n-D  NumberOfTableDimensions=1  BreakpointsForDimension1=time_vector  Table=K_gains(:,5)  ExtrapMethod=Clip  InternalRulePriority=Speed  RndMeth=Simplest
  Mux : Mux  Inputs=5
  K_lqr : Outport
  wires:
  Time/1 -> 1-D Lookup Table2/1, 1-D Lookup Table3/1, 1-D Lookup Table4/1, 1-D Lookup Table1/1, 1-D Lookup Table/1
  1-D Lookup Table4/1 -> Mux/5
  1-D Lookup Table3/1 -> Mux/4
  1-D Lookup Table2/1 -> Mux/3
  1-D Lookup Table1/1 -> Mux/2
  1-D Lookup Table/1 -> Mux/1
  Mux/1 -> K_lqr/1  "K_lqr"

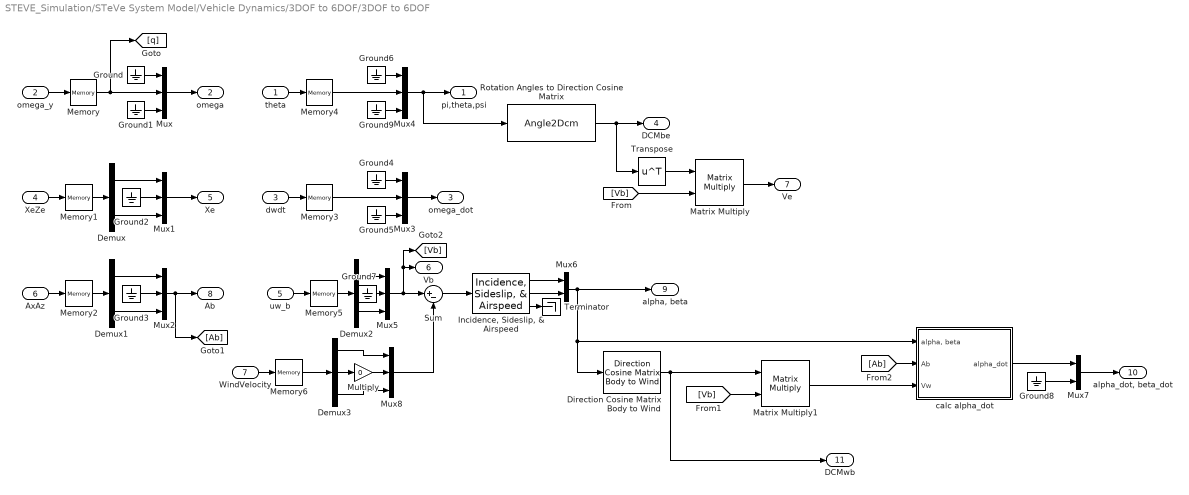
== system STEVE_Simulation/STeVe System Model/Vehicle Dynamics/3DOF to 6DOF/3DOF to 6DOF ==
  theta : Inport
  omega_y : Inport  Port=2
  dwdt : Inport  Port=3
  XeZe : Inport  Port=4
  uw_b : Inport  Port=5
  AxAz : Inport  Port=6
  WindVelocity : Inport  Port=7
  Demux : Demux  Outputs=2
  Demux1 : Demux  Outputs=2
  Demux2 : Demux  Outputs=2
  Demux3 : Demux  Outputs=3
  Direction Cosine Matrix Body to Wind : aerolibtransform2/Direction Cosine Matrix Body to Wind
  Ground{,1..9} (10 alike) : Ground
  "Incidence, Sideslip, & Airspeed" : aerolibasang/Incidence, Sideslip, & Airspeed
  Matrix Multiply : Product  Multiplication=Matrix(*)
  Matrix Multiply1 : Product  Multiplication=Matrix(*)
  Memory{,1..3,5..6} (6 alike) : Memory
  Memory4 : Memory  InitialCondition=Initial.Conditions.theta0
  Multiply : Gain  Gain=0
  Mux{,1..5,8} (7 alike) : Mux  Inputs=3
  Mux6 : Mux  Inputs=2
  Mux7 : Mux  Inputs=2
  Rotation Angles to Direction Cosine Matrix : Angle2Dcm
      settings: AttributesFormatString=Rotation Order: %<rotationOrder>
      mask Display:
      | port_label('input',1,'[R_1,R_2,R_3]','texmode','on')
      | port_label('output',1,'DCM_{be}','texmode','on')
  Sum : Sum  Inputs=|+-
  Terminator : Terminator
  Transpose : Math  Operator=transpose
  calc alpha_dot : Subsystem
  pi,theta,psi : Outport
  omega : Outport  Port=2
  omega_dot : Outport  Port=3
  DCMbe : Outport  Port=4
  Xe : Outport  Port=5
  Vb : Outport  Port=6
  Ve : Outport  Port=7
  Ab : Outport  Port=8
  "alpha, beta" : Outport  Port=9
  "alpha_dot, beta_dot" : Outport  Port=10
  DCMwb : Outport  Port=11
  wires:
  omega_y/1 -> Memory/1
  Memory/1 -> [q], Mux/2
  Ground/1 -> Mux/1
  Ground1/1 -> Mux/3
  Demux/1 -> Mux1/1
  Ground2/1 -> Mux1/2
  Demux/2 -> Mux1/3
  Mux/1 -> omega/1
  XeZe/1 -> Memory1/1
  Memory1/1 -> Demux/1
  Mux1/1 -> Xe/1
  AxAz/1 -> Memory2/1
  Demux1/1 -> Mux2/1
  Demux1/2 -> Mux2/3
  Mux2/1 -> [Ab], Ab/1
  Memory2/1 -> Demux1/1
  Ground3/1 -> Mux2/2
  dwdt/1 -> Memory3/1
  Ground4/1 -> Mux3/1
  Ground5/1 -> Mux3/3
  Mux3/1 -> omega_dot/1
  Memory3/1 -> Mux3/2
  Ground9/1 -> Mux4/3
  Ground6/1 -> Mux4/1
  Mux4/1 -> Rotation Angles to Direction Cosine Matrix/1, pi,theta,psi/1
  theta/1 -> Memory4/1
  Memory4/1 -> Mux4/2
  Rotation Angles to Direction Cosine Matrix/1 -> Transpose/1, DCMbe/1
  Transpose/1 -> Matrix Multiply/1
  [Vb] -> Matrix Multiply/2
  Matrix Multiply/1 -> Ve/1
  uw_b/1 -> Memory5/1
  Demux2/2 -> Mux5/3
  Mux5/1 -> Sum/1, Vb/1, [Vb]
  Demux2/1 -> Mux5/1
  Ground7/1 -> Mux5/2
  Memory5/1 -> Demux2/1
  "Incidence, Sideslip, & Airspeed"/3 -> Terminator/1
  "Incidence, Sideslip, & Airspeed"/1 -> Mux6/1
  "Incidence, Sideslip, & Airspeed"/2 -> Mux6/2
  Mux6/1 -> calc alpha_dot/1("alpha, beta"), Direction Cosine Matrix Body to Wind/1, "alpha, beta"/1
  [Vb] -> Matrix Multiply1/2
  Direction Cosine Matrix Body to Wind/1 -> DCMwb/1, Matrix Multiply1/1
  Matrix Multiply1/1 -> calc alpha_dot/3(Vw)
  [Ab] -> calc alpha_dot/2(Ab)
  calc alpha_dot/1(alpha_dot) -> Mux7/1
  Ground8/1 -> Mux7/2
  Mux7/1 -> "alpha_dot, beta_dot"/1
  Sum/1 -> "Incidence, Sideslip, & Airspeed"/1
  WindVelocity/1 -> Memory6/1
  Memory6/1 -> Demux3/1
  Demux3/1 -> Mux8/1
  Multiply/1 -> Mux8/2
  Demux3/2 -> Multiply/1
  Demux3/3 -> Mux8/3
  Mux8/1 -> Sum/2

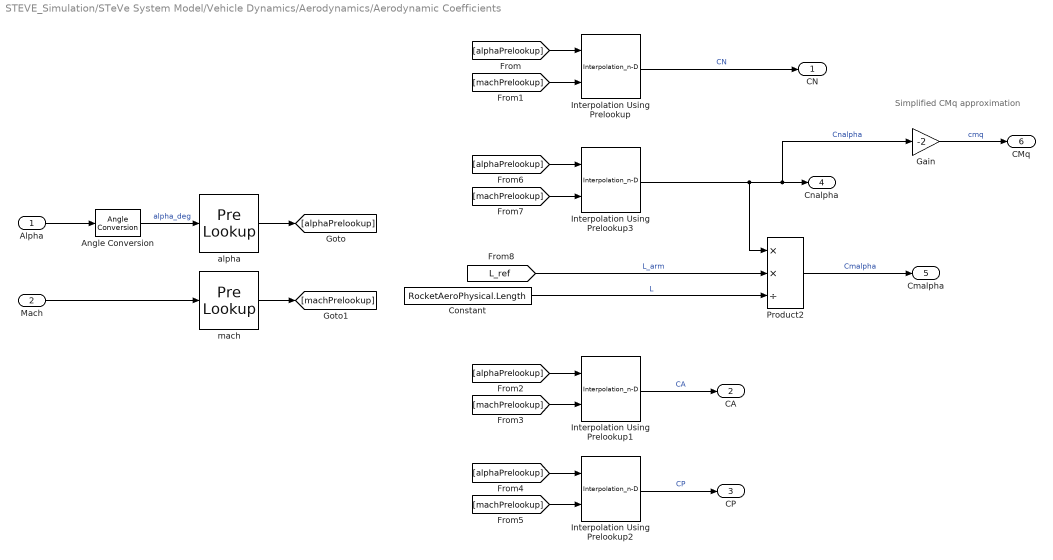
== system STEVE_Simulation/STeVe System Model/Vehicle Dynamics/Aerodynamics/Aerodynamic Coefficients ==
  note: Simplified CMq approximation
  Alpha : Inport
  Mach : Inport  Port=2
  Angle Conversion : aerolibconvert2/Angle Conversion  IU=rad  OU=deg
  Constant : Constant  Value=RocketAeroPhysical.Length
  Gain : Gain  Gain=-2
  Interpolation Using Prelookup : Interpolation_n-D  Table=AeroData.Tables.CN  RequireIndexFractionAsBus=on  InternalRulePriority=Speed
      settings: InputPortMap=u0,u1
  Interpolation Using Prelookup1 : Interpolation_n-D  Table=AeroData.Tables.CAPower_On  RequireIndexFractionAsBus=on  InternalRulePriority=Speed
      settings: InputPortMap=u0,u1
  Interpolation Using Prelookup2 : Interpolation_n-D  Table=AeroData.Tables.CP  RequireIndexFractionAsBus=on  InternalRulePriority=Speed
      settings: InputPortMap=u0,u1
  Interpolation Using Prelookup3 : Interpolation_n-D  Table=AeroData.Tables.Cnalpha  RequireIndexFractionAsBus=on  InternalRulePriority=Speed
      settings: InputPortMap=u0,u1
  Product2 : Product  Inputs=**/
  alpha : PreLookup  BreakpointsData=AeroData.Breakpoints.Alpha  OutputSelection=Index and fraction as bus  IndexSearchMethod=Evenly spaced points  UseLastBreakpoint=on
  mach : PreLookup  BreakpointsData=AeroData.Breakpoints.Mach  OutputSelection=Index and fraction as bus  IndexSearchMethod=Evenly spaced points  ExtrapMethod=Linear
  CN : Outport
  CA : Outport  Port=2
  CP : Outport  Port=3
  Cnalpha : Outport  Port=4
  Cmalpha : Outport  Port=5
  CMq : Outport  Port=6
  wires:
  Interpolation Using Prelookup/1 -> CN/1  "CN"
  alpha/1 -> [alphaPrelookup]
  mach/1 -> [machPrelookup]
  [alphaPrelookup] -> Interpolation Using Prelookup/1
  [machPrelookup] -> Interpolation Using Prelookup/2
  Interpolation Using Prelookup1/1 -> CA/1  "CA"
  [machPrelookup] -> Interpolation Using Prelookup1/2
  [alphaPrelookup] -> Interpolation Using Prelookup1/1
  Interpolation Using Prelookup2/1 -> CP/1  "CP"
  [machPrelookup] -> Interpolation Using Prelookup2/2
  [alphaPrelookup] -> Interpolation Using Prelookup2/1
  Interpolation Using Prelookup3/1 -> Gain/1, Cnalpha/1, Product2/1  "Cnalpha"
  [machPrelookup] -> Interpolation Using Prelookup3/2
  [alphaPrelookup] -> Interpolation Using Prelookup3/1
  Angle Conversion/1 -> alpha/1  "alpha_deg"
  Mach/1 -> mach/1
  Alpha/1 -> Angle Conversion/1
  [L_ref] -> Product2/2  "L_arm"
  Constant/1 -> Product2/3  "L"
  Product2/1 -> Cmalpha/1  "Cmalpha"
  Gain/1 -> CMq/1  "cmq"

== system STEVE_Simulation/STeVe System Model/Vehicle Dynamics/Aerodynamics/DerivedConditions ==
  Speed of sound : Inport
  Air Density : Inport  Port=2
  WindVelocity : Inport  Port=3
  WindAngularRates : Inport  Port=4
  Vb : Inport  Port=5
  Dot Product : DotProduct  OutDataTypeStr=Inherit: Inherit via internal rule
  Dynamic Pressure : aerolibasang/Dynamic Pressure
  Mach Number : aerolibasang/Mach Number
  Saturation : Saturate  UpperLimit=inf  LowerLimit=0
  Sqrt : Sqrt
  Sum : Sum  Inputs=|++
  Mach : Outport
  qbar : Outport  Port=2
  pqrWind : Outport  Port=3
  Airspeed : Outport  Port=4
  wires:
  WindVelocity/1 -> Sum/2
  Vb/1 -> Sum/1
  Speed of sound/1 -> Mach Number/2
  Sum/1 -> Dynamic Pressure/1, Mach Number/1, Dot Product/2, Dot Product/1
  Mach Number/1 -> Mach/1  "Mach"
  Air Density/1 -> Dynamic Pressure/2
  Dynamic Pressure/1 -> qbar/1  "qbar"
  WindAngularRates/1 -> pqrWind/1
  Dot Product/1 -> Saturation/1
  Sqrt/1 -> Airspeed/1
  Saturation/1 -> Sqrt/1
